simulink model "qnetdcmotor"  (R2022b)
settings: Solver=VariableStepAuto  StartTime=0.0  StopTime=10.0  RelTol=1e-3
InitFcn:
  | R = 8.70;
  | Kt = 0.0334;
  | Ke = 0.0334;
  | J = 1.80e-6;
  | L = 0.001;
  | b = 0.000;
settings Model: Creator=Zonularity  LastModifiedBy=Zonularity

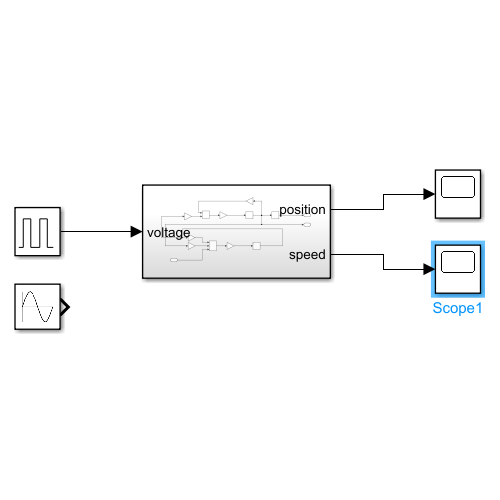
[thumbnail: Simulink's stored preview of the top-level diagram]
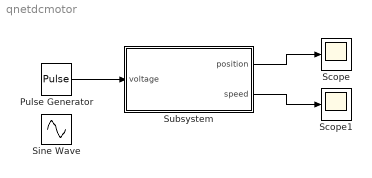
== system qnetdcmotor ==
  Pulse Generator : DiscretePulseGenerator  PulseType=Time based  PulseWidth=50
  Scope : Scope
  Scope1 : Scope
  Sine Wave : Sin  Frequency=3  SampleTime=0
  Subsystem : Subsystem
  wires:
  Subsystem/1(position) -> Scope/1
  Subsystem/2(speed) -> Scope1/1
  Pulse Generator/1 -> Subsystem/1(voltage)

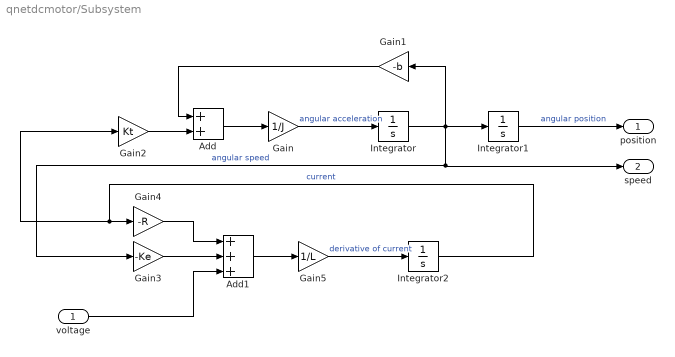
== system qnetdcmotor/Subsystem ==
  voltage : Inport
  Add : Sum
  Add1 : Sum  Inputs=+++
  Gain : Gain  Gain=1/J
  Gain1 : Gain  Gain=-b
  Gain2 : Gain  Gain=Kt
  Gain3 : Gain  Gain=-Ke
  Gain4 : Gain  Gain=-R
  Gain5 : Gain  Gain=1/L
  Integrator : Integrator
  Integrator1 : Integrator
  Integrator2 : Integrator
  position : Outport
  speed : Outport  Port=2
  wires:
  Gain2/1 -> Add/2
  Integrator2/1 -> Gain4/1, Gain2/1  "current"
  Integrator/1 -> speed/1, Gain3/1, Gain1/1, Integrator1/1  "angular speed"
  Add1/1 -> Gain5/1
  voltage/1 -> Add1/3
  Gain3/1 -> Add1/2
  Gain5/1 -> Integrator2/1  "derivative of current"
  Add/1 -> Gain/1
  Gain1/1 -> Add/1
  Gain4/1 -> Add1/1
  Integrator1/1 -> position/1  "angular position"
  Gain/1 -> Integrator/1  "angular acceleration"
